simulink model "Compliance"  (R2020a)
settings: Solver=VariableStepAuto  StartTime=0.0  StopTime=1.0  RelTol=1e-3
values from neighbouring files (symbols this model uses):
  g = 9.81    [params.m]
  KD = diag([  35   45   15    1     0   0])    [params.m]
  KP = diag([ 250  350  100   50     1   1])    [params.m]
libraries: vrlib x1
settings Model: Creator=Sebastiano  LastModifiedBy=Sebastiano

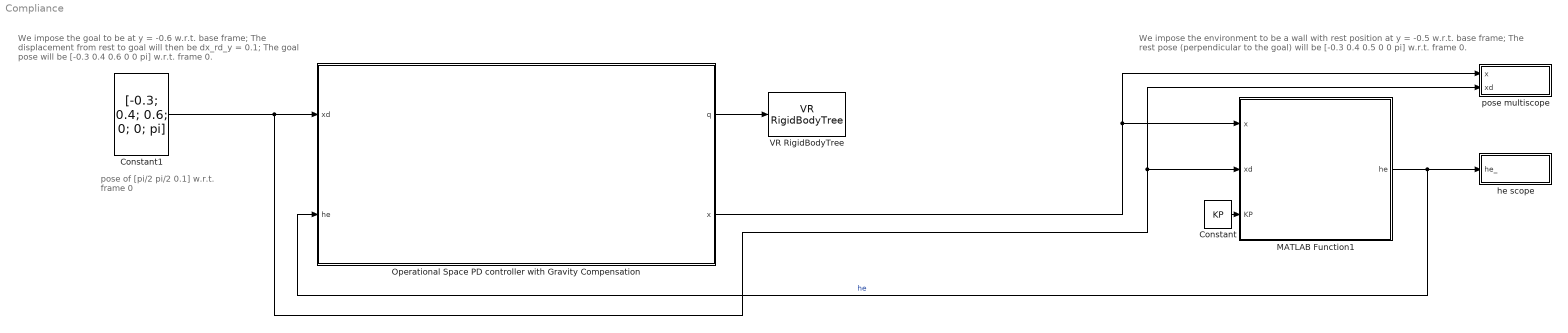
== system Compliance ==
  note: We impose the goal to be at y = -0.6 w.r.t. base frame;
      | The displacement from rest to goal will then be dx_rd_y = 0.1;
      | The goal pose will be [-0.3 0.4 0.6 0 0 pi] w.r.t. frame 0.
  note: We impose the environment to be a wall with rest position at y = -0.5 w.r.t. base frame;
      | The rest pose (perpendicular to the goal) will be [-0.3 0.4 0.5 0 0 pi] w.r.t. frame 0.
  note: pose of [pi/2 pi/2 0.1]
      | w.r.t. frame 0
  Constant : Constant  Value=KP
  Constant1 : Constant  Value=[-0.3; 0.4; 0.6; 0; 0; pi]  VectorParams1D=off
  MATLAB Function1 : MATLAB Function  TreatAsAtomicUnit=on
  Operational Space PD controller with Gravity Compensation : Subsystem
  VR RigidBodyTree : vrlib/VR RigidBodyTree  RBT=robot  useRBT=on  Ts=-1  ForceViewerOpen=on
      settings: SourceProductBaseCode=SL
  he scope : Subsystem
  pose multiscope : Subsystem
  wires:
  Constant1/1 -> MATLAB Function1/2(xd), pose multiscope/2(xd), Operational Space PD controller with Gravity Compensation/1(xd)
  MATLAB Function1/1(he) -> Operational Space PD controller with Gravity Compensation/2(he), he scope/1(he_)  "he"
  Operational Space PD controller with Gravity Compensation/1(q) -> VR RigidBodyTree/1
  Operational Space PD controller with Gravity Compensation/2(x) -> MATLAB Function1/1(x), pose multiscope/1(x)
  Constant/1 -> MATLAB Function1/3(KP)

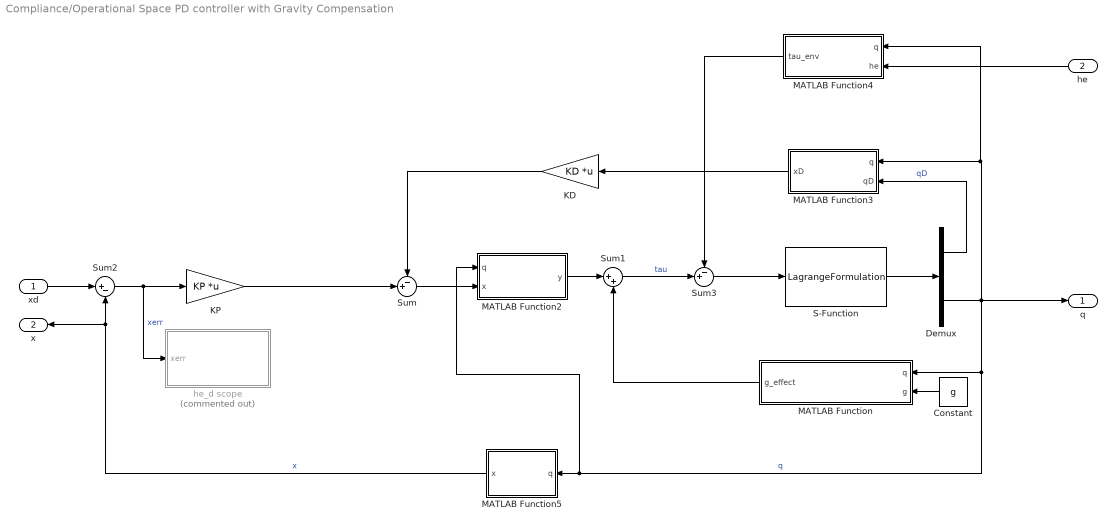
== system Compliance/Operational Space PD controller with Gravity Compensation ==
  xd : Inport
  he : Inport  Port=2
  Constant : Constant  Value=g
  Demux : Demux  Outputs=[3, 3]
  KD : Gain  Gain=KD  Multiplication=Matrix(K*u) (u vector)
  KP : Gain  Gain=KP  Multiplication=Matrix(K*u) (u vector)
  MATLAB Function : MATLAB Function  TreatAsAtomicUnit=on
  MATLAB Function2 : MATLAB Function  TreatAsAtomicUnit=on
  MATLAB Function3 : MATLAB Function  TreatAsAtomicUnit=on
  MATLAB Function4 : MATLAB Function  TreatAsAtomicUnit=on
  MATLAB Function5 : MATLAB Function  TreatAsAtomicUnit=on
  S-Function : S-Function  FunctionName=LagrangeFormulation  Parameters=g  SFunctionDeploymentMode=off  EnableBusSupport=off
  Sum : Sum  Inputs=-+|
  Sum1 : Sum  Inputs=|++
  Sum2 : Sum  Inputs=|+-
  Sum3 : Sum  Inputs=-+|
  he_d scope : Subsystem  Commented=on
  q : Outport
  x : Outport  Port=2
  wires:
  Constant/1 -> MATLAB Function/2(g)
  MATLAB Function3/1(xD) -> KD/1
  Sum/1 -> MATLAB Function2/2(x)
  S-Function/1 -> Demux/1
  KP/1 -> Sum/2
  Sum2/1 -> he_d scope/1(xerr), KP/1  "xerr"
  Demux/1 -> MATLAB Function3/2(qD)  "qD"
  MATLAB Function/1(g_effect) -> Sum1/2
  MATLAB Function5/1(x) -> x/1, Sum2/2  "x"
  Sum3/1 -> S-Function/1
  KD/1 -> Sum/1
  MATLAB Function2/1(y) -> Sum1/1
  Demux/2 -> q/1, MATLAB Function4/1(q), MATLAB Function3/1(q), MATLAB Function2/1(q), MATLAB Function5/1(q), MATLAB Function/1(q)  "q"
  Sum1/1 -> Sum3/2  "tau"
  xd/1 -> Sum2/1
  MATLAB Function4/1(tau_env) -> Sum3/1
  he/1 -> MATLAB Function4/2(he)

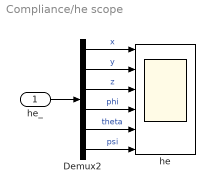
== system Compliance/he scope ==
  he_ : Inport
  Demux2 : Demux  Outputs=[1, 1, 1, 1, 1, 1]
  he : Scope  NumInputPorts=6
  wires:
  Demux2/4 -> he/4  "phi"
  Demux2/3 -> he/3  "z"
  Demux2/6 -> he/6  "psi"
  Demux2/5 -> he/5  "theta"
  Demux2/1 -> he/1  "x"
  he_/1 -> Demux2/1
  Demux2/2 -> he/2  "y"

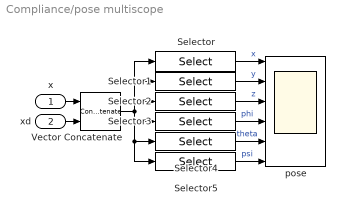
== system Compliance/pose multiscope ==
  x : Inport
  xd : Inport  Port=2
  Selector : Selector  NumberOfDimensions=2  InputPortWidth=3  IndexOptions=Index vector (dialog),Select all  Indices=1,7  OutputSizes=6,6
  Selector1 : Selector  NumberOfDimensions=2  InputPortWidth=3  IndexOptions=Index vector (dialog),Select all  Indices=2,7  OutputSizes=6,6
  Selector2 : Selector  NumberOfDimensions=2  InputPortWidth=3  IndexOptions=Index vector (dialog),Select all  Indices=3,7  OutputSizes=6,6
  Selector3 : Selector  NumberOfDimensions=2  InputPortWidth=3  IndexOptions=Index vector (dialog),Select all  Indices=4,7  OutputSizes=6,6
  Selector4 : Selector  NumberOfDimensions=2  InputPortWidth=3  IndexOptions=Index vector (dialog),Select all  Indices=5,7  OutputSizes=6,6
  Selector5 : Selector  NumberOfDimensions=2  InputPortWidth=3  IndexOptions=Index vector (dialog),Select all  Indices=6,7  OutputSizes=6,6
  Vector Concatenate : Concatenate  Mode=Multidimensional array  ConcatenateDimension=2
  pose : Scope  NumInputPorts=6
  wires:
  x/1 -> Vector Concatenate/1
  xd/1 -> Vector Concatenate/2
  Selector1/1 -> pose/2  "y"
  Selector5/1 -> pose/6  "psi"
  Selector3/1 -> pose/4  "phi"
  Selector/1 -> pose/1  "x"
  Selector4/1 -> pose/5  "theta"
  Vector Concatenate/1 -> Selector/1, Selector1/1, Selector2/1, Selector5/1, Selector4/1, Selector3/1
  Selector2/1 -> pose/3  "z"

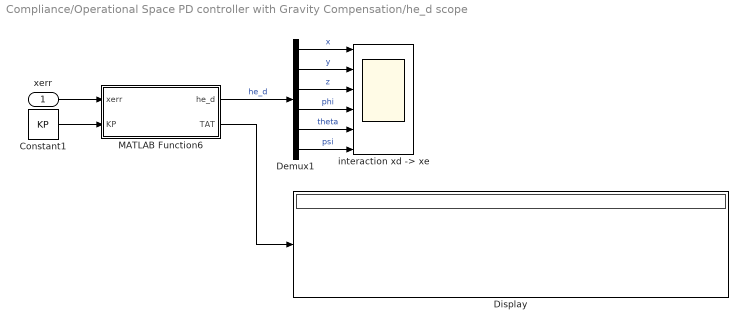
== system Compliance/Operational Space PD controller with Gravity Compensation/he_d scope ==
  xerr : Inport
  Constant1 : Constant  Value=KP
  Demux1 : Demux  Outputs=[1, 1, 1, 1, 1, 1]
  Display : Display
  MATLAB Function6 : MATLAB Function  TreatAsAtomicUnit=on
  "interaction xd -> xe" : Scope  NumInputPorts=6
  wires:
  MATLAB Function6/2(TAT) -> Display/1
  Demux1/6 -> "interaction xd -> xe"/6  "psi"
  Demux1/3 -> "interaction xd -> xe"/3  "z"
  Demux1/4 -> "interaction xd -> xe"/4  "phi"
  Demux1/1 -> "interaction xd -> xe"/1  "x"
  Constant1/1 -> MATLAB Function6/2(KP)
  MATLAB Function6/1(he_d) -> Demux1/1  "he_d"
  xerr/1 -> MATLAB Function6/1(xerr)
  Demux1/5 -> "interaction xd -> xe"/5  "theta"
  Demux1/2 -> "interaction xd -> xe"/2  "y"

== matlab function Compliance/MATLAB Function1 ==
  data: x input; he output; xd input; KP input
function he = environment(x, xd, KP)

% environment params
K = 5*diag([1 1 1 1 1 1]);    % stiffness
wall = 0.5; % constraint position w.r.t. frame 0 (it's y=-0.5 w.r.t. base frame)

if x(3) >= wall  % check is done in frame 0
    % touching the environment! constrained motion
    % set up the rest position frame
    % (basically, same orientation as goal but position is the contact point at the wall)
    xr = x;
    xr(3) = wall;
    xr(4:6) = xd(4:6);
    % calculate the forces
    dx_rd = xd - xr;
    he = (eye(6) + K / KP) \ K * dx_rd;
    dx_ed = KP \ he;
else
    % free motion
    he = zeros(6,1);
    dx_ed = zeros(6,1);
end

he = reshape(he,[6 1]);

== matlab function Compliance/Operational Space PD controller with Gravity Compensation/MATLAB Function ==
  data: q input; g_effect output; g input
function g_effect = gravity(q, g)

g_effect = G_Lagrangian(q, g);

== matlab function Compliance/Operational Space PD controller with Gravity Compensation/MATLAB Function2 ==
  data: q input; y output; x input
function y = JAT(q, x)

y = AnalyticalJacobian(q)' * x;

== matlab function Compliance/Operational Space PD controller with Gravity Compensation/MATLAB Function3 ==
  data: q input; xD output; qD input
function xD = JA(q, qD)

xD = AnalyticalJacobian(q)*qD;

== matlab function Compliance/Operational Space PD controller with Gravity Compensation/MATLAB Function4 ==
  data: q input; he input; tau_env output
function tau_env = J(q, he)

tau_env = Jacobian(q)' * he;

== matlab function Compliance/Operational Space PD controller with Gravity Compensation/MATLAB Function5 ==
  data: q input; x output
function x = K(q)

t1 = q(1);
t2 = q(2);
d3 = q(3);

% wrt frame 0
K = [[ cos(t1 + t2), -sin(t1 + t2), 0, (3*cos(t1 + t2))/10 + (2*cos(t1))/5]
     [ sin(t1 + t2),  cos(t1 + t2), 0, (3*sin(t1 + t2))/10 + (2*sin(t1))/5]
     [            0,             0, 1,                            d3 + 2/5]
     [            0,             0, 0,                                   1]];

pos = K(1:3, 4);
ori = rotm2eul(K(1:3,1:3), 'ZYZ')';

x = [pos; ori];

== matlab function Compliance/Operational Space PD controller with Gravity Compensation/he_d scope/MATLAB Function6 ==
  data: xerr input; he_d output; KP input; TAT output
function [he_d, TAT] = TAinvTKP(xerr, KP)

ori = xerr(4:6);
TAT = TransformAnalitical(ori)';
he_d = TAT \ KP * xerr;
